simulink model "Main_Simulink"  (R2023b)
settings: Solver=FixedStepDiscrete  StartTime=0.0  StopTime=inf  FixedStep=0.001  RelTol=1e-3
undefined symbols (not defined in the file or in its folder): battery_builder_rtmsupport, gcbh, Initial_SOC
libraries: nesl_utility x118, pack_105s34p_structured_lib x105, fl_lib x14, ee_lib x7, dspstat3 x6, BatteryBalancing x1, deeplib x1
(part 9 of 10)

== matlab function Main_Simulink/Battery Management System/Fault Diagnosis System/MATLAB Function3 ==
  data: HVBatCellVltMin input; HVBatCellVltMinV output; HVBatCellVltAvg input
function HVBatCellVltMinV = checkVltMinValidity(HVBatCellVltMin, HVBatCellVltAvg)

% Constants
VLT_THRESHOLD = 1.7;     % Volts
TIME_WINDOW_MS = 100; % 100 ms
TS_MS          = 1;   % fixed step = 1 ms

VALID     = 0;
NOT_VALID = 1;

% Persistent counter (ms)
persistent violationTimeMs

if isempty(violationTimeMs)
    violationTimeMs = 0;
end

% Deviation from average
devMin = abs(HVBatCellVltMin - HVBatCellVltAvg);

% Threshold check
if devMin > VLT_THRESHOLD
    violationTimeMs = violationTimeMs + TS_MS;
else
    violationTimeMs = 0;
end

% Validity decision
if violationTimeMs >= TIME_WINDOW_MS
    HVBatCellVltMinV = NOT_VALID;
else
    HVBatCellVltMinV = VALID;
end

== matlab function Main_Simulink/Battery Management System/Fault Diagnosis System/MATLAB Function ==
  data: HVBatModTempMax input; HVBatModTempMaxV output; HVBatModTempAvg input
function HVBatModTempMaxV = checkTempMaxValidity(HVBatModTempMax, HVBatModTempAvg)

% Constants
TEMP_THRESHOLD = 10;   % degC
TIME_WINDOW_MS = 100;  % 100 ms
TS_MS          = 1;    % fixed step = 1 ms

VALID     = 0;
NOT_VALID = 1;

% Persistent counter (ms)
persistent violationTimeMs

if isempty(violationTimeMs)
    violationTimeMs = 0;
end

% Deviation from average
devMax = abs(HVBatModTempMax - HVBatModTempAvg);

% Threshold check
if devMax > TEMP_THRESHOLD
    violationTimeMs = violationTimeMs + TS_MS;
else
    violationTimeMs = 0;
end

% Validity decision
if violationTimeMs >= TIME_WINDOW_MS
    HVBatModTempMaxV = NOT_VALID;
else
    HVBatModTempMaxV = VALID;
end

== matlab function Main_Simulink/Battery Management System/State of Power Estimation System/Continuus Discharge Power Limits/MATLAB Function1 ==
  data: P2_static input; P2_out output; P2_energy input; P180_kW input
function P2_out  = P2_DeRateSlew(P2_static, P2_energy, P180_kW)
%#codegen
% Computes:
%   P2_target = max(P180_kW, min(P2_static, P2_energy))
% Applies:
%   symmetric slew rate of 1 kW/s (Ts = 0.1 s => 0.1 kW/step)

Ts = 1;                   % [s]
slew_kW_per_s = 1.0;         % [kW/s]
step = slew_kW_per_s * Ts;   % [kW/step] = 0.1

% sanitize
if ~isfinite(P2_static), P2_static = 0; end
if ~isfinite(P2_energy), P2_energy = 0; end
if ~isfinite(P180_kW),   P180_kW   = 0; end

P2_static = max(P2_static, 0);
P2_energy = max(P2_energy, 0);
P180_kW   = max(P180_kW,   0);

% target: apply static + rolling-energy cap, then don't go below continuous
P2_target = min(P2_static, P2_energy);
P2_target = max(P180_kW, P2_target);

% persistent state
persistent P2_prev
if isempty(P2_prev)
    P2_prev = P2_target;   % avoid startup transient
end

% symmetric slew limit
delta = P2_target - P2_prev;

if delta > step
    P2_out = P2_prev + step;
elseif delta < -step
    P2_out = P2_prev - step;
else
    P2_out = P2_target;
end

P2_prev = P2_out;
end

== matlab function Main_Simulink/Battery Management System/Contactor Drive System/MATLAB Function ==
  data: Fault_HVBatRdy input; K1 output; VCU_DriveReady input; VCU_MainHighVltCntctrCmd input; VCU_DC_CntctrCmd input; Sensors_HVBatteryCurrent_BEV input; K2 output; K3 output; K4 output; HVBatCntctrStat output; HVBatCntrWeld_ImpdOpn output; Ke_t_HighVoltageBusActualPrechargeTime output; Ke_I_HighVoltageBusShortageCurrent output; Ke_V_HighVoltagePreChargeThreshold output; Ke_b_WeldCheckEnabler output; Sensors_HVBatteryVoltage_BEV input; Sensors_HVBatteryVoltage_BEV_DCLink input; Sensors_HVBatteryVoltage_BEV_DCFC input; Sensors_HVBatPrecharge_Temp input; Rprecharge input; HVIL_HVBatIntrlk_InternalStat input; VCU_VehSpeed input; HVBatPrechgInbt output; HVBatPrechgInbt input
function [K1, K2, K3, K4, HVBatCntctrStat, HVBatCntrWeld_ImpdOpn, Ke_t_HighVoltageBusActualPrechargeTime, Ke_I_HighVoltageBusShortageCurrent, Ke_V_HighVoltagePreChargeThreshold, Ke_b_WeldCheckEnabler, HVBatPrechgInbt] = fcn(Fault_HVBatRdy, VCU_DriveReady, VCU_MainHighVltCntctrCmd, VCU_DC_CntctrCmd, Sensors_HVBatteryCurrent_BEV, Sensors_HVBatteryVoltage_BEV, Sensors_HVBatteryVoltage_BEV_DCLink, Sensors_HVBatteryVoltage_BEV_DCFC, Sensors_HVBatPrecharge_Temp, Rprecharge, HVIL_HVBatIntrlk_InternalStat, VCU_VehSpeed, HVBatPrechgInbt)
%-----------------------------------------------------------
% McMaster Automotive Resource Centre (MARC)
% Electrical Engineer: Romulo Vieira, M.Sc and MBA - PhD Candidate
%-----------------------------------------------------------
% Purpose: Manage precharge relay and contactor sequence with retry + inhibit logic
%-----------------------------------------------------------
% HVBatCntctrStat Mapping:
% 0 – Idle/Waiting
% 1 – Precharge Active
% 2 – Precharge Complete (Main contactors closed)
% 3 – Precharge Failed (necessary cooldown after unique failures of voltage and current)
% 4 – Inhibit State (necessary cooldown after multiple failures)
% 5 - DCFC Charging
% 6 – Contactor Control Shorted High
% 7 - Contactor Control Shorted Low
% VCU_MainHighVltCntctrCmd mapping:
% 0 - open
% 1 - closed
% 2 - impact_open
% 3 - fast_open
% 7 - invalid
% HVBatCntrWeld_ImpdOpn (Contactor welded and has impeded opening when commanded by BPCM) Mapping:
% 0: Normal
% 1: Stuck_Open
% 2: Stuck_Closed
% 3: SNA
% --- Constants ---
Unset_VbusTargetHitIdx             = -1;   % Flag indicating Vbus threshold not yet hit
Min_Samples                        = 0;    % Minimum number of samples where relays and contactor are both active
% Internal Configuration Parameters
Ke_t_PrechargeFailCoolTime             = 1000;   % Cooldown time after one single failed attempt [ms]
Ke_t_ExtraPrechargeFailCoolPenaltyTime = 1000;   % Additional cooldown after two multiple failures [ms]
Ke_t_PrechargeFailMaxPenalty           = 10000;  % Maximum time threshold before enabling precharge inhibit state
Ke_t_BPCM_Precharge_Fail_Penalty_Time  = 15000;  % Hard inhibit time if failures persist [ms]
Ke_I_HighVoltageBusShortageCurrentMin  = 10.8;   % Minimum expected precharge current [A] (Pack current ≥ 0.6 * (pack voltage / Precharge resistance))
                                                 % // max pack voltage = 450 V, Precharge resistance = 25 ohm
Ke_V_HighVoltagePreChargeThreshold     = 0.98 * Sensors_HVBatteryVoltage_BEV;  % Target voltage threshold
Ke_t_HighVoltageBusPrechargeTime       = 100;    % Maximum allowable time for precharging [ms]
Ke_b_WeldCheckEnabler                  = 1;      % Check if weld check diagnostic is enabled (0 - disabled, 1 - enabled)
Ke_v_WeldCheckEnableSpeed              = 5;      % km/h 
% --- Persistent Variables ---
persistent I_buffer idx HVBatCntctrStat_Aux VbusTargetHitIdx ...
    t_counter last_PrechargeAllw Prchrgpnltytimer PrechargeFailCount last_HVBatCntctrStat_Aux HVBatCntrWeld_ImpdOpn_Aux Ke_b_WeldCheckEnabler_Aux
if isempty(I_buffer)
    I_buffer               = zeros(Ke_t_HighVoltageBusPrechargeTime,1);
    idx                    = 1;
    HVBatCntctrStat_Aux    = 0;
    VbusTargetHitIdx       = Unset_VbusTargetHitIdx;
    t_counter              = 0;
    last_PrechargeAllw     = 0;
    Prchrgpnltytimer       = 0;
    PrechargeFailCount     = 0; % Represented by k_fail in the flowchart
    last_HVBatCntctrStat_Aux = 0;
    HVBatCntrWeld_ImpdOpn_Aux = 0;
    Ke_b_WeldCheckEnabler_Aux = 1;
end
% --- Default Outputs ---
K1 = 0; K2 = 0; K3 = 0; K4 = 0;
HVBatCntctrStat = HVBatCntctrStat_Aux;
Ke_t_HighVoltageBusActualPrechargeTime = 0;
Ke_I_HighVoltageBusShortageCurrent = 0;
%-----------------------------------------------------------
% Weld Check Enable Logic (Explicit & Robust)
%
% Weld check is ENABLED only when:
% - Contactor command is NOT IMPACT_OPEN
% - AND (Contactor command is NOT OPEN
%        OR Vehicle speed <= threshold)
%-----------------------------------------------------------

if VCU_MainHighVltCntctrCmd == 2
    % IMPACT_OPEN → permanently disable weld check
    Ke_b_WeldCheckEnabler_Aux = 0;

elseif (VCU_MainHighVltCntctrCmd == 0) && ...
       (VCU_VehSpeed > Ke_v_WeldCheckEnableSpeed)
    % OPEN + vehicle moving → temporarily disable
    Ke_b_WeldCheckEnabler_Aux = 0;

else
    % All other conditions → weld check allowed
    Ke_b_WeldCheckEnabler_Aux = 1;
end

% FAST_OPEN handling (state reset only)
if VCU_MainHighVltCntctrCmd == 3
    HVBatCntctrStat_Aux = 0;
end

% IMPACT_OPEN must also force state reset
if VCU_MainHighVltCntctrCmd == 2
    HVBatCntctrStat_Aux = 0;
end


% --- State Machine ---
switch HVBatCntctrStat_Aux
    case 0 % OPEN STATE
        % Set the Battery Contactor States
        K1 = 0; K2 = 0; K3 = 0; K4 = 0;
        % Check Initial conditions
        % HVIL_HVBatIntrlk_InternalStat = 1 (pass),
        % HVIL_HVBatIntrlk_InternalStat = 2 (fail)
        % For precharge initiation HVIL_HVBatIntrlk_InternalStat must pass.
        if VCU_MainHighVltCntctrCmd == 1 && HVBatPrechgInbt == 0 && HVIL_HVBatIntrlk_InternalStat == 1 && Fault_HVBatRdy == 1 && VCU_DriveReady == 1 && Sensors_HVBatPrecharge_Temp < 60
            I_buffer(:) = 0;
            idx = 1;
            VbusTargetHitIdx = Unset_VbusTargetHitIdx;
            t_counter = 0;
            HVBatCntctrStat_Aux = 1;
        end

        %% Shorted High
        
        if VCU_MainHighVltCntctrCmd == 0 && Sensors_HVBatteryVoltage_BEV_DCLink > 270 && Ke_b_WeldCheckEnabler_Aux == 1 
            HVBatCntctrStat_Aux = 6;
            HVBatCntrWeld_ImpdOpn_Aux = 2; 
        end

    case 1  % PRECHARGING STATE
        % Abort if initial conditions are no longer valid
        if VCU_MainHighVltCntctrCmd == 0 || HVBatPrechgInbt == 1 || HVIL_HVBatIntrlk_InternalStat == 2 || Fault_HVBatRdy == 0 || VCU_DriveReady == 0 || Sensors_HVBatPrecharge_Temp >= 60
            HVBatCntctrStat_Aux = 0;
        end
        % Set precharge relays ON
        K1 = 0; K2 = 1; K3 = 1; K4 = 0;
        %
        % if Fault_K1_Shorted_Low_Condition == 1
        %     HVBatCntctrStat_Aux = 7; % K1 Shorted Low
        % end
        % if Fault_K4_Shorted_Low_Condition == 1
        %     HVBatCntctrStat_Aux = 7; % K4 Shorted Low
        % end
        % Record current
        if t_counter == 0
            I_buffer(idx) = Sensors_HVBatteryVoltage_BEV / Rprecharge;
        else
            I_buffer(idx) = Sensors_HVBatteryCurrent_BEV;
        end
        Ke_I_HighVoltageBusShortageCurrent = max(I_buffer);
        % Voltage target check
        if VbusTargetHitIdx == Unset_VbusTargetHitIdx && Sensors_HVBatteryVoltage_BEV_DCLink >= Ke_V_HighVoltagePreChargeThreshold
            VbusTargetHitIdx = t_counter + 1;
        end
        % Time since start or since target hit
        if VbusTargetHitIdx ~= Unset_VbusTargetHitIdx
            delta_samples = VbusTargetHitIdx;
        else
            delta_samples = t_counter;
        end
        % SUCCESS - PRECHARGE CONDITIONS ARE MET
        if t_counter < Ke_t_HighVoltageBusPrechargeTime && ...
                VbusTargetHitIdx ~= Unset_VbusTargetHitIdx && delta_samples < Ke_t_HighVoltageBusPrechargeTime && Ke_I_HighVoltageBusShortageCurrent >= Ke_I_HighVoltageBusShortageCurrentMin
            
            % Set the next Battery Contactor Status
            HVBatCntctrStat_Aux = 2;
            % Set the Battery Contactor States
            K1 = 1; K2 = 0; K3 = 0; K4 = 0;
            PrechargeFailCount = 0;
            Prchrgpnltytimer = 0;
        % FAILURE - PRECHARGE CONDITIONS ARE NOT MET
        elseif t_counter == Ke_t_HighVoltageBusPrechargeTime && ...
               (VbusTargetHitIdx == Unset_VbusTargetHitIdx || delta_samples == Ke_t_HighVoltageBusPrechargeTime || Ke_I_HighVoltageBusShortageCurrent < Ke_I_HighVoltageBusShortageCurrentMin)
            % Set the Battery Contactor States
            K1 = 0; K2 = 0; K3 = 0; K4 = 0;
           % Set the Battery Contactor Status
            HVBatCntctrStat_Aux = 3;
            % Update the total cooling time before re-attempt
            PrechargeFailCount = PrechargeFailCount + 1;
            Prchrgpnltytimer = Prchrgpnltytimer + Ke_t_PrechargeFailCoolTime;
            if PrechargeFailCount >= 2
                Prchrgpnltytimer = Ke_t_ExtraPrechargeFailCoolPenaltyTime;
            end
            if PrechargeFailCount >= 10
                HVBatCntctrStat_Aux = 4;
                HVBatPrechgInbt = 1;
                Prchrgpnltytimer = Ke_t_BPCM_Precharge_Fail_Penalty_Time;
            end
        end
        % Update counters
        t_counter = t_counter + 1;
        idx = idx + 1;
        if idx > Ke_t_HighVoltageBusPrechargeTime, idx = 1; end
    case 2  % PRECHARGE COMPLETE OR CLOSED
        % Set the Battery Contactor States
        K1 = 1; K2 = 0; K3 = 0; K4 = 0;
        % If statement to detect DCFC charging
        if VCU_DC_CntctrCmd == 1
            HVBatCntctrStat_Aux = 5; % DCFC CHARGING
        end
        if VCU_MainHighVltCntctrCmd == 0
            HVBatCntctrStat_Aux = 0;
        end

        if VCU_MainHighVltCntctrCmd == 1 && Sensors_HVBatteryVoltage_BEV_DCLink < 270 && Ke_b_WeldCheckEnabler_Aux == 1
            HVBatCntctrStat_Aux = 7;
            HVBatCntrWeld_ImpdOpn_Aux = 1;
        end

    case 3 % FAULT: PRECHARGE FAILED STATE 4 --> 3
        % Set the Battery Contactor States
        K1 = 0; K2 = 0; K3 = 0; K4 = 0;
        if Prchrgpnltytimer > 0
            Prchrgpnltytimer = Prchrgpnltytimer - 1;
        else
            HVBatCntctrStat_Aux = 0;
        end
    case 4  % FAULT: PRECHARGE INHIBIT STATE - 5 -- > 4
        % Set the Battery Contactor States
        K1 = 0; K2 = 0; K3 = 0; K4 = 0;
        if Prchrgpnltytimer > 0
            Prchrgpnltytimer = Prchrgpnltytimer - 1;
        else
            Prchrgpnltytimer = 0;
            HVBatPrechgInbt = 0;
            HVBatCntctrStat_Aux = 0;
            PrechargeFailCount = 0;
        end
    case 5 % DCFC CHARGING
        % Set the Battery Contactor States
        K1 = 1; K2 = 0; K3 = 0; K4 = 1;
        if VCU_DC_CntctrCmd == 0
            if VCU_MainHighVltCntctrCmd == 0
                HVBatCntctrStat_Aux = 0; % switch to OPEN
            else
                HVBatCntctrStat_Aux = 2; % switch to CLOSED
            end
        end
    
    case 6 % FAULT: Shorted High
       
        if VCU_MainHighVltCntctrCmd == 0 && Sensors_HVBatteryVoltage_BEV_DCLink < 270
            HVBatCntctrStat_Aux = 0;
            HVBatCntrWeld_ImpdOpn_Aux = 0;
        end

    case 7 % FAULT: Shorted Low

        if VCU_DC_CntctrCmd == 0 && Sensors_HVBatteryVoltage_BEV_DCFC < 270 && VCU_MainHighVltCntctrCmd == 1 && Sensors_HVBatteryVoltage_BEV_DCLink > 270
            HVBatCntctrStat_Aux = 2;
            HVBatCntrWeld_ImpdOpn_Aux = 0;
        end
    otherwise
        K1 = 0; K2 = 0; K3 = 0; K4 = 0;
        HVBatCntctrStat_Aux = 0;
end
% --- Final Outputs ---
HVBatCntctrStat = HVBatCntctrStat_Aux;
HVBatCntrWeld_ImpdOpn = HVBatCntrWeld_ImpdOpn_Aux;
Ke_b_WeldCheckEnabler = Ke_b_WeldCheckEnabler_Aux;
Ke_t_HighVoltageBusActualPrechargeTime = max(0, VbusTargetHitIdx + ...
    Min_Samples * (VbusTargetHitIdx ~= Unset_VbusTargetHitIdx));
last_PrechargeAllw = double(Fault_HVBatRdy);
last_HVBatCntctrStat_Aux = HVBatCntctrStat_Aux;
end

== matlab function Main_Simulink/Battery Management System/Fault Diagnosis System/MATLAB Function1 ==
  data: HVBatModTempMin input; HVBatModTempMinV output; HVBatModTempAvg input
function HVBatModTempMinV = checkTempMinValidity(HVBatModTempMin, HVBatModTempAvg)

% Constants
TEMP_THRESHOLD = 10;   % degC
TIME_WINDOW_MS = 100;  % 100 ms
TS_MS          = 1;    % fixed step = 1 ms

VALID     = 0;
NOT_VALID = 1;

% Persistent counter (ms)
persistent violationTimeMs

if isempty(violationTimeMs)
    violationTimeMs = 0;
end

% Deviation from average
devMin = abs(HVBatModTempMin - HVBatModTempAvg);

% Threshold check
if devMin > TEMP_THRESHOLD
    violationTimeMs = violationTimeMs + TS_MS;
else
    violationTimeMs = 0;
end

% Validity decision
if violationTimeMs >= TIME_WINDOW_MS
    HVBatModTempMinV = NOT_VALID;
else
    HVBatModTempMinV = VALID;
end

== matlab function Main_Simulink/Battery Management System/State of Power Estimation System/Continuus Discharge Power Limits/MATLAB Function3 ==
  data: P10_static input; P10_out output; P10_energy input; P180_kW input
function P10_out  = P10_DeRateSlew(P10_static, P10_energy, P180_kW)
%#codegen
% Computes:
%   P10_target = max(P180_kW, min(P10_static, P10_energy))
% Applies:
%   symmetric slew rate of 1 kW/s (Ts = 0.1 s => 0.1 kW/step)

Ts = 1;                   % [s]
slew_kW_per_s = 1.0;         % [kW/s]
step = slew_kW_per_s * Ts;   % [kW/step] = 0.1

% sanitize
if ~isfinite(P10_static), P10_static = 0; end
if ~isfinite(P10_energy), P10_energy = 0; end
if ~isfinite(P180_kW),   P180_kW   = 0; end

P10_static = max(P10_static, 0);
P10_energy = max(P10_energy, 0);
P180_kW   = max(P180_kW,   0);

% target: apply static + rolling-energy cap, then don't go below continuous
P10_target = min(P10_static, P10_energy);
P10_target = max(P180_kW, P10_target);

% persistent state
persistent P10_prev
if isempty(P10_prev)
    P10_prev = P10_target;   % avoid startup transient
end

% symmetric slew limit
delta = P10_target - P10_prev;

if delta > step
    P10_out = P10_prev + step;
elseif delta < -step
    P10_out = P10_prev - step;
else
    P10_out = P10_target;
end

P10_prev = P10_out;
end

== matlab function Main_Simulink/Battery Management System/State of Power Estimation System/Continuus Discharge Power Limits/MATLAB Function4 ==
  data: P30_static input; P30_out output; P30_energy input; P180_kW input
function P30_out  = P30_DeRateSlew(P30_static, P30_energy, P180_kW)
%#codegen
% Computes:
%   P30_target = max(P180_kW, min(P30_static, P30_energy))
% Applies:
%   symmetric slew rate of 1 kW/s (Ts = 0.1 s => 0.1 kW/step)

Ts = 1;                   % [s]
slew_kW_per_s = 1.0;         % [kW/s]
step = slew_kW_per_s * Ts;   % [kW/step] = 0.1

% sanitize
if ~isfinite(P30_static), P30_static = 0; end
if ~isfinite(P30_energy), P30_energy = 0; end
if ~isfinite(P180_kW),   P180_kW   = 0; end

P30_static = max(P30_static, 0);
P30_energy = max(P30_energy, 0);
P180_kW   = max(P180_kW,   0);

% target: apply static + rolling-energy cap, then don't go below continuous
P30_target = min(P30_static, P30_energy);
P30_target = max(P180_kW, P30_target);

% persistent state
persistent P30_prev
if isempty(P30_prev)
    P30_prev = P30_target;   % avoid startup transient
end

% symmetric slew limit
delta = P30_target - P30_prev;

if delta > step
    P30_out = P30_prev + step;
elseif delta < -step
    P30_out = P30_prev - step;
else
    P30_out = P30_target;
end

P30_prev = P30_out;
end

== matlab function Main_Simulink/Battery Management System/State of Power Estimation System/Continuus Discharge Power Limits/MATLAB Function5 ==
  data: Pt_kW input; P2_energy output; P10_energy output; P30_energy output; P180_kW input; E150_G output; E170_G output; E178_G output; E180_G output
function [P2_energy, P10_energy, P30_energy, E150_G, E170_G, E178_G, E180_G] = rollingEnergy_multi(Pt_kW, P180_kW)
%#codegen

% ---- configuration ----
Ts     = 1;                 % sample time [s]
Ts_h   = Ts/3600.0;         % seconds -> hours

% Window lengths for Ts = 1 s
N178   = 178;
N170   = 170;
N150   = 150;

T180_h = 180/3600.0;        % 180 s in hours

% Precompute once (compile-time constants)
inv_dth_2h  = 1800.0;       % 3600/2
inv_dth_10h =  360.0;       % 3600/10
inv_dth_30h =  120.0;       % 3600/30

% Clamp Pt_kW to >= 0 (cheaper than max() on many targets)
if Pt_kW < 0
    Pt_kW = 0;
end

% ---- persistent state (one circular buffer per window) ----
persistent buf178 idx178 cnt178 E178_kWh ...
           buf170 idx170 cnt170 E170_kWh ...
           buf150 idx150 cnt150 E150_kWh ...
           ramp2_active cap2_ramp ...
           ramp10_active cap10_ramp ...
           ramp30_active cap30_ramp

if isempty(idx178)
    % rolling buffers / integrators
    buf178 = zeros(N178,1); idx178 = 1; cnt178 = 0; E178_kWh = 0.0;
    buf170 = zeros(N170,1); idx170 = 1; cnt170 = 0; E170_kWh = 0.0;
    buf150 = zeros(N150,1); idx150 = 1; cnt150 = 0; E150_kWh = 0.0;

    % ramp state (kept, though not used unless you uncomment ramp section)
    ramp2_active  = false; cap2_ramp  = 0.0;
    ramp10_active = false; cap10_ramp = 0.0;
    ramp30_active = false; cap30_ramp = 0.0;
end

% -------- 178 s window fed by Pt_kW (for 2 s cap) --------
Pold = 0.0;
if cnt178 < N178
    cnt178 = cnt178 + 1;              % warm-up
else
    Pold = buf178(idx178);            % oldest sample leaving
end
buf178(idx178) = Pt_kW;
idx178 = idx178 + 1; if idx178 > N178, idx178 = 1; end
E178_kWh = E178_kWh + (Pt_kW - Pold) * Ts_h;  % kWh

% -------- 170 s window fed by Pt_kW (for 10 s cap) --------
Pold = 0.0;
if cnt170 < N170
    cnt170 = cnt170 + 1;
else
    Pold = buf170(idx170);
end
buf170(idx170) = Pt_kW;
idx170 = idx170 + 1; if idx170 > N170, idx170 = 1; end
E170_kWh = E170_kWh + (Pt_kW - Pold) * Ts_h;

% -------- 150 s window fed by Pt_kW (for 30 s cap) --------
Pold = 0.0;
if cnt150 < N150
    cnt150 = cnt150 + 1;
else
    Pold = buf150(idx150);
end
buf150(idx150) = Pt_kW;
idx150 = idx150 + 1; if idx150 > N150, idx150 = 1; end
E150_kWh = E150_kWh + (Pt_kW - Pold) * Ts_h;

% ---- 180 s energy budget (kWh) from P180_kW ----
E180_kWh = P180_kW * T180_h;

% ---- Remaining Energy (kW) - For each time horizon ----
dE = E180_kWh - E178_kWh;
if dE < 0, dE = 0; end
P2_energy = dE * inv_dth_2h;

dE = E180_kWh - E170_kWh;
if dE < 0, dE = 0; end
P10_energy = dE * inv_dth_10h;

dE = E180_kWh - E150_kWh;
if dE < 0, dE = 0; end
P30_energy = dE * inv_dth_30h;

% ---- start ramps when each window first fills ----
if (~ramp2_active)  && (cnt178 >= N178)
    ramp2_active = true;  cap2_ramp  = P2_energy;
end
if (~ramp10_active) && (cnt170 >= N170)
    ramp10_active = true; cap10_ramp = P10_energy;
end
if (~ramp30_active) && (cnt150 >= N150)
    ramp30_active = true; cap30_ramp = P30_energy;
end

% ---- outputs ----
E150_G = E150_kWh;
E170_G = E170_kWh;
E178_G = E178_kWh;
E180_G = E180_kWh;

end

== matlab function Main_Simulink/Battery Management System/State of Power Estimation System/Continuus Charge Power Limits/MATLAB Function1 ==
  data: P2_static input; P2_out output; P2_energy input; P180_kW input
function P2_out  = P2_DeRateSlew(P2_static, P2_energy, P180_kW)
%#codegen
% Computes:
%   P2_target = max(P180_kW, min(P2_static, P2_energy))
% Applies:
%   symmetric slew rate of 1 kW/s (Ts = 0.1 s => 0.1 kW/step)

Ts = 1;                   % [s]
slew_kW_per_s = 1.0;         % [kW/s]
step = slew_kW_per_s * Ts;   % [kW/step] = 0.1

% sanitize
if ~isfinite(P2_static), P2_static = 0; end
if ~isfinite(P2_energy), P2_energy = 0; end
if ~isfinite(P180_kW),   P180_kW   = 0; end

P2_static = max(P2_static, 0);
P2_energy = max(P2_energy, 0);
P180_kW   = max(P180_kW,   0);

% target: apply static + rolling-energy cap, then don't go below continuous
P2_target = min(P2_static, P2_energy);
P2_target = max(P180_kW, P2_target);

% persistent state
persistent P2_prev
if isempty(P2_prev)
    P2_prev = P2_target;   % avoid startup transient
end

% symmetric slew limit
delta = P2_target - P2_prev;

if delta > step
    P2_out = P2_prev + step;
elseif delta < -step
    P2_out = P2_prev - step;
else
    P2_out = P2_target;
end

P2_prev = P2_out;
end

== matlab function Main_Simulink/Battery Management System/Contactor Drive System/AC Plug In Charging ==
  settings: updateMethod=DISCRETE
  data: HVBat_DC_CntctrStat output; VCU_DCChargeInitialized input; VCU_MainHighVltCntctrCmd input; VCU_ChargingSysSts input; VCU_Charger_Plugin_Status input; Fault_HVBatCell_Voltage_High_Thrsh input; Fault_HVBatRdy input; Sensors_HVBatModTempMax input; Sensors_HVBatCellVltMax input; Sensors_HVBatSOCMax input; Cntctr_K1 input; Cntctr_K2 input; Cntctr_K3 input; HVBatChargeStat output; MaxChargeCurrentAllowed output; MaxChargeRegenPowerAllowed output; HVBatMaxCellVltAlld output; HVBatMaxPkVltAllwd output
function [HVBat_DC_CntctrStat, HVBatChargeStat, MaxChargeCurrentAllowed, MaxChargeRegenPowerAllowed, HVBatMaxCellVltAlld, HVBatMaxPkVltAllwd] = ac( ...
    VCU_DCChargeInitialized, VCU_MainHighVltCntctrCmd, VCU_ChargingSysSts, VCU_Charger_Plugin_Status, ...
    Fault_HVBatCell_Voltage_High_Thrsh, Fault_HVBatRdy, ...
    Sensors_HVBatModTempMax, Sensors_HVBatCellVltMax, Sensors_HVBatSOCMax, Cntctr_K1, Cntctr_K2, Cntctr_K3)

% ===========================
%% INPUTS
% Time - Current time (s)
% VCU_MainHighVltCntctrCmd - VCU command for main contactor (0/1/2/3/7)
% Cntctr_K3,Cntctr_K2,Cntctr_K1 - Physical contactor feedbacks (1=closed, 0=open)
% Fault_HVBatRdy - Fault flag (0=Fault, 1=Ok)
% VCU_ChargingSysSts - 0=Not Charging,1=Charging,2=Interrupted,3=Complete
% VCU_Charger_Plugin_Status - 0=Unplugged, 1=Plugged
% Fault_HVBatCell_Voltage_High_Thrsh - Max allowable cell voltage (V)
% Sensors_HVBatModTempMax, Sensors_HVBatCellVltMax, Sensors_HVBatSOCMax - vectors
% VDC - DC bus voltage (V)
% HVBatMaxPkVltAllwd 
% HVBatMaxCellVltAlld

%% OUTPUTS
% HVBat_DC_CntctrStat - 0=Open, 1=Closed, 2=Faulted
% HVBatChargeStat     - 0=Not Ready, 1=Ready, 2=Charging, 3=Fault, 6=Complete
% MaxChargeCurrentAllowed - Allowed charging current (A)
% P_charge            - Estimated DC charging power (W)

%% --- Lookup Table for Max Charge Current [SOC vs Temp] ---
SOC = [0 5 10 15 20 25 30 35 40 45 50 55 60 65 70 75 80 85 90 95 100]; % 19 + 2 points
Temp = [-25 -20 -10 0 5 10 20 25 35 40 50]; % 11 points

ACChgCurrentProfile = [ ...
  0.05 0.05 0.05 0.05 0.05 0.05 0.05 0.05 0.05 0.05 0.05 0.05 0.05 0.02 0.02 0.01 0.01 0.01 0.01 0.01 0.00; ...
  0.06 0.06 0.06 0.06 0.06 0.06 0.06 0.06 0.06 0.06 0.06 0.06 0.06 0.02 0.02 0.02 0.02 0.01 0.01 0.01 0.00; ...
  0.45 0.45 0.45 0.45 0.45 0.15 0.15 0.15 0.15 0.09 0.09 0.09 0.09 0.03 0.03 0.03 0.03 0.02 0.02 0.02 0.00; ...
  0.70 0.70 0.70 0.70 0.70 0.70 0.70 0.70 0.70 0.50 0.50 0.50 0.50 0.25 0.25 0.25 0.25 0.10 0.10 0.09 0.00; ...
  0.85 0.85 0.85 0.85 0.85 0.85 0.85 0.85 0.85 0.75 0.75 0.75 0.75 0.63 0.63 0.58 0.44 0.35 0.24 0.12 0.00; ...
  0.88 0.88 0.88 0.88 0.88 0.88 0.88 0.88 0.88 0.88 0.88 0.88 0.88 0.88 0.88 0.68 0.59 0.35 0.24 0.12 0.00; ...
  0.88 0.88 0.88 0.88 0.88 0.88 0.88 0.88 0.88 0.88 0.88 0.88 0.88 0.88 0.88 0.88 0.74 0.59 0.44 0.29 0.00; ...
  0.88 0.88 0.88 0.88 0.88 0.88 0.88 0.88 0.88 0.88 0.88 0.88 0.88 0.88 0.88 0.88 0.88 0.74 0.59 0.44 0.00; ...
  0.88 0.88 0.88 0.88 0.88 0.88 0.88 0.88 0.88 0.88 0.88 0.88 0.88 0.88 0.88 0.88 0.88 0.74 0.65 0.59 0.00; ...
  0.88 0.88 0.88 0.88 0.88 0.88 0.88 0.88 0.88 0.88 0.88 0.88 0.88 0.88 0.88 0.88 0.88 0.76 0.74 0.60 0.00; ...
  0.88 0.88 0.88 0.88 0.88 0.88 0.88 0.88 0.88 0.88 0.88 0.88 0.88 0.88 0.88 0.88 0.88 0.60 0.60 0.48 0.00 ...
];

%% --- Calibrations ---
persistent Ke_t_DCFC_CntctrOpn Ke_T_HighChrgTempThresholdIn Ke_T_LowChrgTempThresholdIn ...
           Ke_U_ChargeCompletionVlt ...
           ParallelCellNum Ke_t_ChargeCompletionHold HVBatChargeTimer ...
           chargeCompleteFlag overTempFlag
if isempty(Ke_t_DCFC_CntctrOpn)
    Ke_t_DCFC_CntctrOpn = 1500;     % milliseconds      
    Ke_T_HighChrgTempThresholdIn = 50;   
    Ke_T_LowChrgTempThresholdIn  = -25;  
    Ke_U_ChargeCompletionVlt = 4.14;     
    ParallelCellNum = 34;
    Ke_t_ChargeCompletionHold = 300;     % milliseconds
    HVBatChargeTimer = 0;
    chargeCompleteFlag = false;
    overTempFlag = false;
end


persistent Ke_RegenVltMargin Ke_P_MaxChargeRegen
if isempty(Ke_RegenVltMargin)
    Ke_RegenVltMargin   = 0.05;   % [V] margin below Fault_HVBatCell_Voltage_High_Thrsh
    Ke_P_MaxChargeRegen = 11000;  % [W] max allowed regen during charge
end

%% --- Persistent states ---
persistent HVBatChargeStat_Aux MaxChargeCurrentAllowed_Aux MaxChargeRegenPowerAllowed_Aux
if isempty(HVBatChargeStat_Aux)
    HVBatChargeStat_Aux = 0;
    MaxChargeCurrentAllowed_Aux = 0;
    MaxChargeRegenPowerAllowed_Aux = 0;
end

%% Default outputs 
HVBatChargeStat = HVBatChargeStat_Aux;
MaxChargeCurrentAllowed = MaxChargeCurrentAllowed_Aux;
MaxChargeRegenPowerAllowed = MaxChargeRegenPowerAllowed_Aux;

%% --- AC Plug-in readiness
ready_cond = (VCU_DCChargeInitialized == 0) && (VCU_Charger_Plugin_Status == 1) && ~chargeCompleteFlag && ~overTempFlag;
main_contactor_ok = (VCU_MainHighVltCntctrCmd == 1) && (Cntctr_K1 == 1) && (Cntctr_K2 == 0) && (Cntctr_K3 == 0);

if ready_cond
    if main_contactor_ok && Fault_HVBatRdy == 1
        HVBatChargeStat_Aux = 1; % Ready
    else
        HVBatChargeStat_Aux = 0; % Not Ready
    end
elseif VCU_Charger_Plugin_Status == 1 && chargeCompleteFlag
    HVBatChargeStat_Aux = 6; % Complete
else
    HVBatChargeStat_Aux = 0; % Not Ready
end
MaxChargeCurrentAllowed_Aux = 0;
MaxChargeRegenPowerAllowed_Aux = 0;

%% Charging logic
Temp_actual = Sensors_HVBatModTempMax;
SOC_actual  = Sensors_HVBatSOCMax;
Vmax = Sensors_HVBatCellVltMax;

handshake_ok = (HVBatChargeStat_Aux == 1 && VCU_ChargingSysSts == 1);
if handshake_ok
    HVBatChargeStat_Aux = 2; % charge allow current
    if ~chargeCompleteFlag && ~overTempFlag && Temp_actual < Ke_T_HighChrgTempThresholdIn && Temp_actual > Ke_T_LowChrgTempThresholdIn && Vmax < Ke_U_ChargeCompletionVlt
        MaxChargeCurrentAllowed_Aux = ParallelCellNum * interp2(SOC, Temp, ACChgCurrentProfile, SOC_actual, Temp_actual);
    end
end

%% --- Charge Completion
if (HVBatChargeStat_Aux == 2) && ...
       (VCU_ChargingSysSts == 1 || VCU_ChargingSysSts == 3) && ...
       (Vmax >= Ke_U_ChargeCompletionVlt) && ...
       (~chargeCompleteFlag) && ...
       (~overTempFlag)
    if HVBatChargeTimer < 0
        HVBatChargeTimer = 0;
    end
    HVBatChargeTimer = HVBatChargeTimer + 1;
    if HVBatChargeTimer >= Ke_t_ChargeCompletionHold
        HVBatChargeStat_Aux = 6;
        MaxChargeCurrentAllowed_Aux = 0;
        MaxChargeRegenPowerAllowed_Aux = 0;
        chargeCompleteFlag = true;
    end
else
    HVBatChargeTimer = -1;
end

%% --- Overtemperature
if Temp_actual >= Ke_T_HighChrgTempThresholdIn || Temp_actual <= Ke_T_LowChrgTempThresholdIn
    HVBatChargeStat_Aux = 3;
    MaxChargeCurrentAllowed_Aux = 0;
    MaxChargeRegenPowerAllowed_Aux = 0;
    overTempFlag = true;
elseif overTempFlag && Temp_actual <= (Ke_T_HighChrgTempThresholdIn - 5) && Temp_actual >= (Ke_T_LowChrgTempThresholdIn + 5)
    overTempFlag = false;
end

%% --- Regen Power Limit
if VCU_ChargingSysSts == 1
    if Vmax >= Fault_HVBatCell_Voltage_High_Thrsh
        % No regen allowed at or above max allowable cell voltage
        MaxChargeCurrentAllowed_Aux = 0;
        MaxChargeRegenPowerAllowed_Aux = 0;
    
    elseif Vmax >= (Fault_HVBatCell_Voltage_High_Thrsh - Ke_RegenVltMargin)
        % Linearly reduce regen as voltage approaches limit
        scale = (Fault_HVBatCell_Voltage_High_Thrsh - Vmax) / Ke_RegenVltMargin;
        MaxChargeRegenPowerAllowed_Aux = max(0, scale * Ke_P_MaxChargeRegen);
    
    else
        % Full regen allowed (charge-mode limited)
        MaxChargeRegenPowerAllowed_Aux = Ke_P_MaxChargeRegen;
    end
end

% Fault handling
if (VCU_ChargingSysSts == 1 && Fault_HVBatRdy == 0)
    HVBatChargeStat_Aux = 3;
    MaxChargeCurrentAllowed_Aux = 0;
    MaxChargeRegenPowerAllowed_Aux = 0;
end

%% Overvoltage handling
if Vmax > Fault_HVBatCell_Voltage_High_Thrsh
    HVBatChargeStat_Aux = 3;
    MaxChargeCurrentAllowed_Aux = 0;
    MaxChargeRegenPowerAllowed_Aux = 0;
end

%% Reset completion flag ONLY when unplugged
if VCU_Charger_Plugin_Status == 0
    chargeCompleteFlag = false;
end

%% Outputs
HVBatChargeStat = HVBatChargeStat_Aux;
MaxChargeCurrentAllowed = MaxChargeCurrentAllowed_Aux;
MaxChargeRegenPowerAllowed = MaxChargeRegenPowerAllowed_Aux;
if isnan(MaxChargeCurrentAllowed), MaxChargeCurrentAllowed = 0; end
if isnan(MaxChargeRegenPowerAllowed), MaxChargeRegenPowerAllowed = 0; end

%% --- Step 3: Update Max Voltages
HVBatMaxCellVltAlld = Fault_HVBatCell_Voltage_High_Thrsh;
HVBatMaxPkVltAllwd = Fault_HVBatCell_Voltage_High_Thrsh * 105; % example for 105 series cells

%% DC Contactor state will always be open
HVBat_DC_CntctrStat = 0;

end

== matlab function Main_Simulink/Battery Management System/State of Power Estimation System/Continuus Charge Power Limits/MATLAB Function3 ==
  data: P10_static input; P10_out output; P10_energy input; P180_kW input
function P10_out  = P10_DeRateSlew(P10_static, P10_energy, P180_kW)
%#codegen
% Computes:
%   P10_target = max(P180_kW, min(P10_static, P10_energy))
% Applies:
%   symmetric slew rate of 1 kW/s (Ts = 0.1 s => 0.1 kW/step)

Ts = 1;                   % [s]
slew_kW_per_s = 1.0;         % [kW/s]
step = slew_kW_per_s * Ts;   % [kW/step] = 0.1

% sanitize
if ~isfinite(P10_static), P10_static = 0; end
if ~isfinite(P10_energy), P10_energy = 0; end
if ~isfinite(P180_kW),   P180_kW   = 0; end

P10_static = max(P10_static, 0);
P10_energy = max(P10_energy, 0);
P180_kW   = max(P180_kW,   0);

% target: apply static + rolling-energy cap, then don't go below continuous
P10_target = min(P10_static, P10_energy);
P10_target = max(P180_kW, P10_target);

% persistent state
persistent P10_prev
if isempty(P10_prev)
    P10_prev = P10_target;   % avoid startup transient
end

% symmetric slew limit
delta = P10_target - P10_prev;

if delta > step
    P10_out = P10_prev + step;
elseif delta < -step
    P10_out = P10_prev - step;
else
    P10_out = P10_target;
end

P10_prev = P10_out;
end

== matlab function Main_Simulink/Battery Management System/Cell Balancing System/MATLAB Function2 ==
  data: isBalancingActive_Curr input; BalStat output; BalStat_Prev input
function BalStat = balancingStatus(isBalancingActive_Curr, BalStat_Prev)

% Default: hold previous state
BalStat = BalStat_Prev;

if isBalancingActive_Curr == 1
    % Balancing currently active
    BalStat = 1;

elseif isBalancingActive_Curr == 0
    if BalStat_Prev == 1
        % Transition from active → inactive
        BalStat = 2;   % Completed
    elseif BalStat_Prev == 0 || BalStat_Prev == 2
        % Remain inactive or completed
        BalStat = BalStat_Prev;
    end
end

end

== matlab function Main_Simulink/Battery Management System/State of Power Estimation System/Continuus Charge Power Limits/MATLAB Function4 ==
  data: P30_static input; P30_out output; P30_energy input; P180_kW input
function P30_out  = P30_DeRateSlew(P30_static, P30_energy, P180_kW)
%#codegen
% Computes:
%   P30_target = max(P180_kW, min(P30_static, P30_energy))
% Applies:
%   symmetric slew rate of 1 kW/s (Ts = 0.1 s => 0.1 kW/step)

Ts = 1;                   % [s]
slew_kW_per_s = 1.0;         % [kW/s]
step = slew_kW_per_s * Ts;   % [kW/step] = 0.1

% sanitize
if ~isfinite(P30_static), P30_static = 0; end
if ~isfinite(P30_energy), P30_energy = 0; end
if ~isfinite(P180_kW),   P180_kW   = 0; end

P30_static = max(P30_static, 0);
P30_energy = max(P30_energy, 0);
P180_kW   = max(P180_kW,   0);

% target: apply static + rolling-energy cap, then don't go below continuous
P30_target = min(P30_static, P30_energy);
P30_target = max(P180_kW, P30_target);

% persistent state
persistent P30_prev
if isempty(P30_prev)
    P30_prev = P30_target;   % avoid startup transient
end

% symmetric slew limit
delta = P30_target - P30_prev;

if delta > step
    P30_out = P30_prev + step;
elseif delta < -step
    P30_out = P30_prev - step;
else
    P30_out = P30_target;
end

P30_prev = P30_out;
end

== matlab function Main_Simulink/Battery Management System/State of Power Estimation System/Continuus Charge Power Limits/MATLAB Function5 ==
  data: Pt_kW input; P2_energy output; P10_energy output; P30_energy output; P180_kW input; E150_G output; E170_G output; E178_G output; E180_G output
function [P2_energy, P10_energy, P30_energy, E150_G, E170_G, E178_G, E180_G] = rollingEnergy_multi(Pt_kW, P180_kW)
%#codegen

% ---- configuration ----
Ts     = 1;                 % sample time [s]
Ts_h   = Ts/3600.0;         % seconds -> hours

% Window lengths for Ts = 1 s
N178   = 178;
N170   = 170;
N150   = 150;

T180_h = 180/3600.0;        % 180 s in hours

% Precompute once (compile-time constants)
inv_dth_2h  = 1800.0;       % 3600/2
inv_dth_10h =  360.0;       % 3600/10
inv_dth_30h =  120.0;       % 3600/30

% Clamp Pt_kW to >= 0 (cheaper than max() on many targets)
if Pt_kW < 0
    Pt_kW = 0;
end

% ---- persistent state (one circular buffer per window) ----
persistent buf178 idx178 cnt178 E178_kWh ...
           buf170 idx170 cnt170 E170_kWh ...
           buf150 idx150 cnt150 E150_kWh ...
           ramp2_active cap2_ramp ...
           ramp10_active cap10_ramp ...
           ramp30_active cap30_ramp

if isempty(idx178)
    % rolling buffers / integrators
    buf178 = zeros(N178,1); idx178 = 1; cnt178 = 0; E178_kWh = 0.0;
    buf170 = zeros(N170,1); idx170 = 1; cnt170 = 0; E170_kWh = 0.0;
    buf150 = zeros(N150,1); idx150 = 1; cnt150 = 0; E150_kWh = 0.0;

    % ramp state (kept, though not used unless you uncomment ramp section)
    ramp2_active  = false; cap2_ramp  = 0.0;
    ramp10_active = false; cap10_ramp = 0.0;
    ramp30_active = false; cap30_ramp = 0.0;
end

% -------- 178 s window fed by Pt_kW (for 2 s cap) --------
Pold = 0.0;
if cnt178 < N178
    cnt178 = cnt178 + 1;              % warm-up
else
    Pold = buf178(idx178);            % oldest sample leaving
end
buf178(idx178) = Pt_kW;
idx178 = idx178 + 1; if idx178 > N178, idx178 = 1; end
E178_kWh = E178_kWh + (Pt_kW - Pold) * Ts_h;  % kWh

% -------- 170 s window fed by Pt_kW (for 10 s cap) --------
Pold = 0.0;
if cnt170 < N170
    cnt170 = cnt170 + 1;
else
    Pold = buf170(idx170);
end
buf170(idx170) = Pt_kW;
idx170 = idx170 + 1; if idx170 > N170, idx170 = 1; end
E170_kWh = E170_kWh + (Pt_kW - Pold) * Ts_h;

% -------- 150 s window fed by Pt_kW (for 30 s cap) --------
Pold = 0.0;
if cnt150 < N150
    cnt150 = cnt150 + 1;
else
    Pold = buf150(idx150);
end
buf150(idx150) = Pt_kW;
idx150 = idx150 + 1; if idx150 > N150, idx150 = 1; end
E150_kWh = E150_kWh + (Pt_kW - Pold) * Ts_h;

% ---- 180 s energy budget (kWh) from P180_kW ----
E180_kWh = P180_kW * T180_h;

% ---- Remaining Energy (kW) - For each time horizon ----
dE = E180_kWh - E178_kWh;
if dE < 0, dE = 0; end
P2_energy = dE * inv_dth_2h;

dE = E180_kWh - E170_kWh;
if dE < 0, dE = 0; end
P10_energy = dE * inv_dth_10h;

dE = E180_kWh - E150_kWh;
if dE < 0, dE = 0; end
P30_energy = dE * inv_dth_30h;

% ---- start ramps when each window first fills ----
if (~ramp2_active)  && (cnt178 >= N178)
    ramp2_active = true;  cap2_ramp  = P2_energy;
end
if (~ramp10_active) && (cnt170 >= N170)
    ramp10_active = true; cap10_ramp = P10_energy;
end
if (~ramp30_active) && (cnt150 >= N150)
    ramp30_active = true; cap30_ramp = P30_energy;
end

% ---- outputs ----
E150_G = E150_kWh;
E170_G = E170_kWh;
E178_G = E178_kWh;
E180_G = E180_kWh;

end

== matlab function Main_Simulink/Battery Management System/Cell Balancing System/MATLAB Function3 ==
  data: HVBatModTempMax input; BalancingEnabled output; HVBatChargeStat input
function BalancingEnabled = balancingEnabled(HVBatModTempMax, HVBatChargeStat)
if HVBatModTempMax < 65 && HVBatChargeStat == 2
    BalancingEnabled = 1;
else
    BalancingEnabled = 0;
end

== matlab function Main_Simulink/Battery Management System/State of Charge Estimation System/MATLAB Function ==
  data: MinCellSOC input; MaxCellSOC input; HVBatSOC output
function HVBatSOC = fcn(MinCellSOC, MaxCellSOC)

SOCMaxLimit = 100;
SOCMinLimit = 0;

MidPoint = (MaxCellSOC + MinCellSOC)/2;

UpperMid = SOCMaxLimit - ((MaxCellSOC - MinCellSOC)/2);

LowerMid = SOCMinLimit + ((MaxCellSOC - MinCellSOC)/2);

% Base the weight factor for max and min cell soc on location of midpoint
LowWeightNum = (UpperMid - MidPoint);

LowWeightDen = max((UpperMid - LowerMid),1e-6);

% Update the weight used to determine how important the min cell soc will be
LowWeight = LowWeightNum / LowWeightDen;

if LowWeight < 0 
    LowWeight = 0;
elseif LowWeight > 1
    LowWeight = 1;
else
    LowWeight = LowWeightNum / LowWeightDen;
end

% Update the weight used to determine how important the max cell soc will be

HighWeight = 1 - LowWeight;

HVBatSOC = HighWeight*MaxCellSOC + LowWeight*MinCellSOC;

== matlab function Main_Simulink/Battery Management System/State of Charge Estimation System/For Each Subsystem1/MATLAB Function8 ==
  data: SOC input; SOC_Output output
function SOC_Output = Denormalize(SOC)

Max.Output = 1.003127354307489;
Min.Output = 0;
SOC_Output = SOC*(Max.Output-Min.Output) + Min.Output;

== matlab function Main_Simulink/Battery Management System/State of Charge Estimation System/For Each Subsystem1/Subsystem/Extended Kalman Filter ==
  data: Current input; zSOC output; Voltage input; Temperature input; x input; P input; xf output; P1 output; R0 input; R1 input; R2 input; R3 input; C1 input; C2 input; C3 input; R input; Q1 input; Q2 input; Q3 input; Q4 input; Capacity_Ah input
function [zSOC,xf,P1] = EKF(Current,Voltage,Temperature, x,P, R0, R1, R2, R3, C1, C2, C3, R, Q1, Q2, Q3, Q4, Capacity_Ah)
dt=1;
Cn= Capacity_Ah * 3600;
eta=1/Cn;

if Temperature > 35 
Uocv_Poly = [155.308726440546	-597.267889991014	941.407823927130	-786.245252453370	374.778019277070	-101.680174572827	15.4391438256495	2.44338048778122];
% If the temperature is 30 degrees - Use the appropriate model
elseif Temperature <= 35 && Temperature > 25
Uocv_Poly = [138.928430420310	-542.186837887723	871.684367149938	-746.949184290739	367.246636435314	-102.941810495874	15.9644846135961	2.43390736885817];
elseif Temperature <= 25 && Temperature > 15 
Uocv_Poly = [41.9907040354371	-146.371215697789	208.983468492983	-161.903644094484	76.3799686156644	-22.9174190685987	5.03882959997569	2.96993144460831];
% If the temperature is 10 degrees - Use the appropriate model
elseif Temperature <= 15 &&  Temperature > 5
Uocv_Poly = [41.3582787879049	-159.555903843513	258.269521427887	-229.239317160976	121.034268329469	-38.0364814483066	7.52554750623064	2.80926945740385];
% If the temperature is 0 degrees - Use the appropriate model
elseif Temperature <= 5 &&  Temperature > -5
Uocv_Poly = [65.2104799744181	-231.270325870870	330.835554425856	-248.541714354954	108.184344633976	-28.7430805632201	5.56626748675298	2.92542882347389];
% If the temperature is n10 degrees - Use the appropriate model    
elseif Temperature <= -5 &&  Temperature > -12
Uocv_Poly = [155.428533819214	-625.876064954366	1049.49643519607	-945.462920784072	491.150026602732	-146.223151851062	23.9095547800117	1.77398485767751];
% If the temperature is n20 degrees - Use the appropriate model        
else
Uocv_Poly = [897.736834678282	-4025.58216179188	7586.06189168444	-7774.74541179878	4673.36306827772	-1646.23270590737	315.576035521964	-21.9823984511360];
end
    
%% EXTENDED KALMAN FILTER
Q=diag([Q1 Q2 Q3 Q4]); % covariance of process
R=R;        % covariance of measurement  0.1

%%
curr=Current;
z = Voltage;     % measurments

  f=@(x)[( 1-dt/(R1*C1) )*x(1)+dt*curr/C1;...
       ( 1-dt/(R2*C2) )*x(2)+dt*curr/C2;...
       ( 1-dt/(R3*C3) )*x(3)+dt*curr/C3;...
       x(4)-dt*eta*curr];  % Nonlinear equations - Kalman Filter

  h=@(x) polyval(Uocv_Poly,x(4))  -x(1)-x(2)-x(3)-curr*R0; % Measurement equations - Kalman Filter

[xf,P1] = ekf1(f,x,P,h,z,Q,R);
xV_e = xf ;                           % save states
zSOC=xV_e(4,1);                             %SOC

%zV_e  = h_fun(xf);                          % save voltage estimated
function [x,P,V_error]=ekf1(f,x,P,h,z,Q,R)
% EKF   Extended Kalman Filter for nonlinear dynamic systems
% [x, P] = ekf(f,x,P,h,z,Q,R) returns state estimate, x and state covariance, P 
% for nonlinear dynamic system:
%           x_k+1 = f(x_k) + w_k
%           z_k   = h(x_k) + v_k
% where w ~ N(0,Q) meaning w is gaussian noise with covariance Q
%       v ~ N(0,R) meaning v is gaussian noise with covariance R
% Inputs:   f: function handle for f(x)
%           x: "a priori" state estimate
%           P: "a priori" estimated state covariance
%           h: fanction handle for h(x)
%           z: current measurement
%           Q: process noise covariance 
%           R: measurement noise covariance
% Output:   x: "a posteriori" state estimate
%           P: "a posteriori" state covariance
%

[x2,A]=jaccsd1(f,x);    %nonlinear update and linearization at current state
P=A*P*A'+Q;                 %partial update
[z1,H]=jaccsd2(h,x2);    %nonlinear measurement and linearization
P12=P*H';                   %cross covariance
%%%%%% was comented
%     K=P12*inv(H*P12+R);               %Kalman filter gain
%     x=x1+K*(z-z1);                    %state estimate
%     P=P-K*P12';                       %state covariance matrix
%%%%%%    
R=chol(H*P12+R);            %Cholesky factorization
U=P12/R;                    %K=U/R'; Faster because of back substitution
x=x2+U*(R'\(z-z1));         %Back substitution to get state update
V_error=z-z1;
P=P-U*U';                   %Covariance update, U*U'=P12/R/R'*P12'=K*P12.


% function [F_val]=F_fun(xf1)
% F_val=[( 1-dt/(R1*C1) )*xf1(1)+dt*curr/C1;...
%        ( 1-dt/(R2*C2) )*xf1(2)+dt*curr/C2;...
%        ( 1-dt/(R3*C3) )*xf1(3)+dt*curr/C3;...
%        xf1(4)-dt*eta*curr];  % nonlinear state equations
% end


function [z,A]=jaccsd1(f,x3)
% JACCSD Jacobian through complex step differentiation
            % [z J] = jaccsd(f,x)
            % z = f(x)
            % J = f'(x)
%
z=f(x3);
n=numel(x3);
m=numel(z);
A=zeros(m,n);
h1=n*eps;
x1=ones(n,1).*complex(n,1);
for k=1:n
    x1=x3;
    x1(k)=(x1(k)+h1*i);
    A(:,k)=imag(f(x1))/h1;
end
end


function [z,A]=jaccsd2(h, x3)
% JACCSD Jacobian through complex step differentiation
            % [z J] = jaccsd(f,x)
            % z = f(x)
            % J = f'(x)
z=h(x3);
n=numel(x3);
m=numel(z);
A=zeros(m,n);
h1=n*eps;
x1=ones(n,1).*complex(n,1);
for k=1:n
    x1=x3;
    x1(k)=(x1(k)+h1*i);
    xx=h(x1);
    A(:,k)=imag(xx)/h1;
end
end


end
end

== matlab function Main_Simulink/Battery Management System/Contactor Drive System/MATLAB Function1 ==
  data: DCChargeInitialized input; MaxChargeCurrentAllowed_AC input; output output; MaxChargeCurrentAllowed_DC input
function output = fcn(DCChargeInitialized, MaxChargeCurrentAllowed_AC, MaxChargeCurrentAllowed_DC)
    if DCChargeInitialized == 0
        output = MaxChargeCurrentAllowed_AC;
    else
        output = MaxChargeCurrentAllowed_DC;
    end

== matlab function Main_Simulink/Battery Management System/Contactor Drive System/MATLAB Function2 ==
  data: DCChargeInitialized input; HVBatChargeStat_AC input; output output; HVBatChargeStat_DC input
function output = fcn(DCChargeInitialized, HVBatChargeStat_AC, HVBatChargeStat_DC)
    if DCChargeInitialized == 0
        output = HVBatChargeStat_AC;
    else
        output = HVBatChargeStat_DC;
    end

== matlab function Main_Simulink/Battery Management System/Contactor Drive System/MATLAB Function3 ==
  data: DCChargeInitialized input; HVBat_DC_CntctrStat_AC input; output output; HVBat_DC_CntctrStat_DC input
function output = fcn(DCChargeInitialized, HVBat_DC_CntctrStat_AC, HVBat_DC_CntctrStat_DC)
    if DCChargeInitialized == 0
        output = HVBat_DC_CntctrStat_AC;
    else
        output = HVBat_DC_CntctrStat_DC;
    end
